simulink model "VehicleDynamics3D"  (R2017a)
settings: Solver=ode15s  StartTime=0.0  StopTime=StopTime  FixedStep=.001  MaxStep=maxStep  RelTol=relTol  AbsTol=absTol  EnableMultiTasking=on
PreLoadFcn:
  | VehicleDynamicsInitialization
model workspace: external: MATLAB File sm_suspension_templates_params.m (data not in the file)
values from neighbouring files (symbols this model uses):
  followerCameraX = 7.5    [VehicleDynamicsInitialization.m]
  followerCameraZ = 3    [VehicleDynamicsInitialization.m]
  frontCameraX = -1.75    [VehicleDynamicsInitialization.m]
  frontCameraZ = 0.35    [VehicleDynamicsInitialization.m]
  isoCameraAimX = (1/2)*wheelbase    (= 0.75)    [VehicleDynamicsInitialization.m]
  isoCameraX = -3.1    [VehicleDynamicsInitialization.m]
  isoCameraY = 3.5    [VehicleDynamicsInitialization.m]
  isoCameraZ = 1.5    [VehicleDynamicsInitialization.m]
  Load = 200    [VehicleDynamicsInitialization.m]
  maxSteeringDisplacement = 10    [VehicleDynamicsInitialization.m]
  minSteeringDisplacement = -10    [VehicleDynamicsInitialization.m]
  SetPaceSampleTime = 0.1    [VehicleDynamicsInitialization.m]
  steeringInput = 0    [VehicleDynamicsInitialization.m]
  vehicleSpeed_kph = 0    [VehicleDynamicsInitialization.m]
  wheelbase = 1.5    [VehicleDynamicsInitialization.m]
undefined symbols (not defined in the file or in its folder): dwb, Floor, sigbuilder_block, wheel, X, Y, Z
libraries: sm_lib x195, sm_suspension_templates_lib x34, nesl_utility x15, Contact_Forces_Lib x4, simulink x2, fl_lib x1, aerolibanimutils x1
(part 5 of 7)

== system VehicleDynamics3D/RearSuspension/L Spr-Damp Assm ==
  Cyl Bracket : sm_suspension_templates_lib/Single Bracket  L=Lb  W=Wb  T=Tb  Rh=Rbh  rho=rho  clr=cclr
  Cyl Bracket XForm : sm_lib/Frames and Transforms/Rigid Transform  TranslationMethod=StandardAxis  TranslationStandardOffset=Lc/2  TranslationLengthUnit=cm  TranslationStandardAxis=-Z  TranslationCartesianOffset=[0 0 0]  TranslationROffset=0  TranslationROffsetUnits=m  TranslationZOffset=0  TranslationZOffsetUnits=m  TranslationThetaOffset=0  TranslationThetaOffsetUnits=deg  RotationMethod=AlignedAxes  RotationAngleUnits=deg  RotationStandardAxis=+Z  RotationAngle=0  RotationArbitraryAxis=[0 0 1]  FollAlignAxisA=+Z  BaseAlignAxisA=-Z  FollAlignAxisB=+X  BaseAlignAxisB=-X  RotationSequenceAxes=FollowerAxes  RotationSequence=XYX  RotationSequenceAngles=[0 0 0]  RotationSequenceAnglesUnits=deg  RotationMatrix=[1 0 0; 0 1 0; 0 0 1]
  Cyl-Piston Joint : sm_lib/Joints/Prismatic Joint  SenseConstraintForce=off  SenseConstraintForceX=off  SenseConstraintForceY=off  SenseConstraintForceZ=off  SenseConstraintTorque=off  SenseConstraintTorqueX=off  SenseConstraintTorqueY=off  SenseConstraintTorqueZ=off  SenseTotalForce=off  SenseTotalForceX=off  SenseTotalForceY=off  SenseTotalForceZ=off  SenseTotalTorque=off  SenseTotalTorqueX=off  SenseTotalTorqueY=off  SenseTotalTorqueZ=off  CompositeWrenchDir=FollowerOnBase  CompositeWrenchFrame=BaseFrame  EquilibriumPosition=Ls-(Lc-Lp)/2  EquilibriumPositionUnits=cm  SpringStiffness=Ks  SpringStiffnessUnits=N/m  DampingCoefficient=Kb  DampingCoefficientUnits=N/(m/s)  TorqueActuationMode=NoTorque  MotionActuationMode=ComputedMotion  SensePosition=on  SenseVelocity=off  SenseAcceleration=off  SenseTorqueForce=off  PositionTargetSpecify=off  PositionTargetPriority=Low  PositionTargetValue=Lp/2  PositionTargetValueUnits=cm  VelocityTargetSpecify=off  VelocityTargetPriority=High  VelocityTargetValue=0  VelocityTargetValueUnits=m/s
  Cylinder : sm_lib/Body Elements/Solid  InertiaType=CalculateFromGeometry  Mass=1  MassUnits=kg  CenterOfMass=[0 0 0]  CenterOfMassUnits=m  MomentsOfInertia=[1 1 1]  MomentsOfInertiaUnits=kg*m^2  ProductsOfInertia=[0 0 0]  ProductsOfInertiaUnits=kg*m^2  DensityBased=on  Density=rho  DensityUnits=kg/(m^3)  DoExposeReferenceFrame=on  SerializedFrames=<Frames/>  GraphicType=FromGeometry  MarkerShape=Sphere  MarkerSize=10  MarkerSizeUnits=m  GraphicVisPropType=SimpleVisualProperties  GraphicDiffuseColor=cclr  GraphicSpecularColor=[0.5 0.5 0.5 1.0]  GraphicAmbientColor=[0.15 0.15 0.15 1.0]  GraphicEmissiveColor=[0.0 0.0 0.0 1.0]  GraphicShininess=75  GraphicOpacity=0.75  GeometryShape=GeneralSolidOfRevolution  RectangleSize=[1 1]  RectangleSizeUnits=m  BrickDimensions=[1 1 1]  BrickDimensionUnits=m  CylinderRadius=1  CylinderRadiusUnits=m  CylinderLength=1  CylinderLengthUnits=m  SphereRadius=1  SphereRadiusUnits=m  EllipsoidRadii=[1 1 1]  EllipsoidRadiiUnits=m  ExtrusionCrossSection=[1 1; -1 1; -1 -1; 1 -1]  ExtrusionCrossSectionUnits=m  ExtrusionLength=1  ExtrusionLengthUnits=m  PolygonNumSides=3  PolygonOuterRadius=1  PolygonOuterRadiusUnits=m  ExtGeomFileType=STL  ExtGeomFileUnits=m  RevolutionCrossSection=cyl_xsec  RevolutionCrossSectionUnits=cm  RevolutionExtent=Full  RevolutionAngle=180  RevolutionAngleUnits=deg
  PS-Simulink Converter : nesl_utility/PS-Simulink Converter  PhysicalDomain=network_engine_domain  SubClassName=ps_output  LeftPortType=input  RightPortType=output  PseudoPeriodic=off  Frequencies=[]  Unit=cm  AffineConversion=off
  Pistion Bracket : sm_suspension_templates_lib/Single Bracket  L=Lb  W=Wb  T=Tb  Rh=Rbh  rho=rho  clr=pclr
  Piston : sm_lib/Body Elements/Solid  InertiaType=CalculateFromGeometry  Mass=1  MassUnits=kg  CenterOfMass=[0 0 0]  CenterOfMassUnits=m  MomentsOfInertia=[1 1 1]  MomentsOfInertiaUnits=kg*m^2  ProductsOfInertia=[0 0 0]  ProductsOfInertiaUnits=kg*m^2  DensityBased=on  Density=rho  DensityUnits=kg/(m^3)  DoExposeReferenceFrame=on  SerializedFrames=<Frames/>  GraphicType=FromGeometry  MarkerShape=Sphere  MarkerSize=10  MarkerSizeUnits=m  GraphicVisPropType=SimpleVisualProperties  GraphicDiffuseColor=pclr  GraphicSpecularColor=[0.5 0.5 0.5 1.0]  GraphicAmbientColor=[0.15 0.15 0.15 1.0]  GraphicEmissiveColor=[0.0 0.0 0.0 1.0]  GraphicShininess=75  GraphicOpacity=1  GeometryShape=GeneralSolidOfRevolution  RectangleSize=[1 1]  RectangleSizeUnits=m  BrickDimensions=[1 1 1]  BrickDimensionUnits=m  CylinderRadius=1  CylinderRadiusUnits=m  CylinderLength=1  CylinderLengthUnits=m  SphereRadius=1  SphereRadiusUnits=m  EllipsoidRadii=[1 1 1]  EllipsoidRadiiUnits=m  ExtrusionCrossSection=[1 1; -1 1; -1 -1; 1 -1]  ExtrusionCrossSectionUnits=m  ExtrusionLength=1  ExtrusionLengthUnits=m  PolygonNumSides=3  PolygonOuterRadius=1  PolygonOuterRadiusUnits=m  ExtGeomFileType=STL  ExtGeomFileUnits=m  RevolutionCrossSection=piston_xsec  RevolutionCrossSectionUnits=cm  RevolutionExtent=Full  RevolutionAngle=180  RevolutionAngleUnits=deg
  Piston Bracket XForm : sm_lib/Frames and Transforms/Rigid Transform  TranslationMethod=StandardAxis  TranslationStandardOffset=Lp/2  TranslationLengthUnit=cm  TranslationStandardAxis=+Z  TranslationCartesianOffset=[0 0 0]  TranslationROffset=0  TranslationROffsetUnits=m  TranslationZOffset=0  TranslationZOffsetUnits=m  TranslationThetaOffset=0  TranslationThetaOffsetUnits=deg  RotationMethod=None  RotationAngleUnits=deg  RotationStandardAxis=+Z  RotationAngle=0  RotationArbitraryAxis=[0 0 1]  FollAlignAxisA=+Z  BaseAlignAxisA=+Z  FollAlignAxisB=+X  BaseAlignAxisB=-X  RotationSequenceAxes=FollowerAxes  RotationSequence=XYX  RotationSequenceAngles=[0 0 0]  RotationSequenceAnglesUnits=deg  RotationMatrix=[1 0 0; 0 1 0; 0 0 1]
  Terminator : Terminator
  P : PMIOPort  Port=1  Side=Right
  C : PMIOPort  Port=2  Side=Left
  wires:
  PS-Simulink Converter/1 -> Terminator/1  "RLSuspensionTravel_cm"
  connections:
  C/RConn1 -- Cyl Bracket/LConn1
  Pistion Bracket/LConn1 -- P/RConn1
  Pistion Bracket/RConn1 -- Piston Bracket XForm/RConn1
  Cyl Bracket/RConn1 -- Cyl Bracket XForm/RConn1
  Cyl-Piston Joint/RConn1 -- Piston/RConn1 -- Piston Bracket XForm/LConn1
  Cylinder/RConn1 -- Cyl-Piston Joint/LConn1 -- Cyl Bracket XForm/LConn1
  Cyl-Piston Joint/RConn2 -- PS-Simulink Converter/LConn1

== system VehicleDynamics3D/RearSuspension/L Suspension Assembly ==
  Knuckle : Subsystem  mask(Steering knuckle){H=dwb.knuckle.height, L=dwb.knuckle.length, T=dwb.knuckle.thickness, Wpr=dwb.knuckle.wheelattachprojwidth, Hpr=dwb.knuckle.wheelattachprojheight, Wc=dwb.knuckle.wishboneconnectorwidth, Rd=dwb.knuckle.driveshaftradius, Hd=dwb.knuckle.driveshaftheight, Rr=dwb.knuckle.chamferradius, Rt=dwb.knuckle.transitionradius, Rb=dwb.knuckle.ball.radius, Rp=dwb.knuckle.pin.radius, Hp=dwb.knuckle.pin.height, Ls=dwb.knuckle.steerarm.length, Ws=dwb.knuckle.steerarm.width, Ts=dwb.knuckle.steerarm.thickness, Hsf=dwb.knuckle.steerarm.forkheight, Lsf=dwb.knuckle.steerarm.forklength, Osf=dwb.knuckle.steerarm.forkoffset, Rsp=dwb.knuckle.pinradius, Rsr=dwb.knuckle.chamferradius, Rev=on, rho=dwb.knuckle.density, clr=dwb.knuckle.color}
      mask prompts: H "Height (cm):"; L "Length (cm):"; T "Thickness (cm):"; Wpr "Width of wheel attach projection (cm):"; Hpr "Height of wheel attach projection (cm):"; Wc "Width of wishbone connectors (cm):"; Rd "Drive shaft hole radius (cm):"; Hd "Drive shaft bearing housing height (cm):"; Rr "Chamfer/fillet radius (cm):"; Rt "Transition radius to wheel attach projection (cm):"; Rb "Ball radius (cm):"; Rp "Pin radius (cm):"; Hp "Pin height (cm):"; Ls "Length of arm (cm):"; Ws "Width of arm (cm):"; Ts "Thickness of arm (cm):"; Hsf "Height of forked section (cm):"; Lsf "Length of forked section (cm):"; Osf "Offset of forked section (cm):"; Rsp "Pin radius (cm):"; Rsr "Chamfer/fillet radius (cm):"; Rev "Reverse direction:"; rho "Density (kg/m^3):"; clr "Color ([r g b]):"
      mask help: This block models a steering knuckle. The wheel hub attaches to the steering knuckle. The steering knuckle attaches to the wishbone links. The ports U and D correspond to the frames where the knuckle connects to the wishbone links. The port W corresponds to the frame where the wheel hub attaches to the knuckle. The knuckle also has a rigidly attached steering arm that attaches to the steering rack via tie rods. The port S corresponds to the frame where the steering arm attaches to the tie rod.
      mask init:
      | s_knuckle_xsec = [0 -Hd/2; 0 -Hpr/2; Wpr -Hpr/2; Wpr -H/2;
      |                 Wpr+Wc -H/2; Wpr+Wc -H/2+T; Wpr+T -H/2+T;
      |                  Wpr+T -Hd/2];
      | 
      | s_knuckle_xsec = simmechanics.demohelpers.round_corners(s_knuckle_xsec, 2:7, ...
      |                              [Rr Rt Rr*ones(1,4)], 20);
      | 
      | n_knuckle_xsec = flipud([s_knuckle_xsec(:,1) -s_knuckle_xsec(:,2)]);                         
      | 
      | Roh = sqrt((L/2)^2 + (Hd/2)^2);
      | phi = atan2(Hd,L);
      | theta = linspace(pi/2-phi,pi/2+phi,50)';
      | sh_xsec = [Roh*cos(theta) Roh*sin(theta)];
      | theta = linspace(3*pi/2-phi,3*pi/2+phi,50)';
      | sh_xsec = [sh_xsec; Roh*cos(theta) Roh*sin(theta)];
      | theta = linspace(5*pi/2-phi,pi/2-phi,100)';
      | sh_xsec = [sh_xsec; sh_xsec(1,:); Rd*cos(theta) Rd*sin(theta)];
      | 
      | % Convert Rev variable into +/- 1 instead of 0 or 1
      | sgn = (2*Rev-1);
      mask Display:
      | image(imread(fullfile(matlabroot,'toolbox','physmod','sm','smdemos','suspension_templates','images','sm_isuspension_knuckle.png')));
      | port_label('RConn',1,'U');
      | port_label('RConn',2,'D');
      | port_label('LConn',1,'W');
  Lower Wishbone : sm_suspension_templates_lib/Lower Wishbone  L1=dwb.lwb.longlength  L2=dwb.lwb.shortlength  L3=dwb.lwb.wheellinklength  W3=dwb.lwb.wheellinkwidth  W=dwb.lwb.width  T=dwb.lwb.thickness  Rb=dwb.lwb.baseradius  Ob=dwb.lwb.basearcoffset  Rev=on  Lb=dwb.lwb.bracket.length  Rsh=dwb.lwb.bracket.radius  Rs=dwb.lwb.socket.radius  Hi=dwb.lwb.socket.height  Rh=dwb.lwb.socket.holeradius  Oh=dwb.lwb.socket.holeoffset  Odb=dwb.lwb.damperbracket.offset  Wdb=dwb.lwb.damperbracket.width  Ldb=dwb.lwb.damperbracket.length  Tdb=dwb.lwb.damperbracket.thickness  Sdb=dwb.lwb.damperbracket.spacing  Rhdb=dwb.lwb.damperbracket.holeradius  rho=dwb.lwb.density  clr=dwb.lwb.color
  SW Damp Joint : sm_lib/Joints/Revolute Joint  SenseConstraintForce=off  SenseConstraintForceX=off  SenseConstraintForceY=off  SenseConstraintForceZ=off  SenseConstraintTorque=off  SenseConstraintTorqueX=off  SenseConstraintTorqueY=off  SenseConstraintTorqueZ=off  SenseTotalForce=off  SenseTotalForceX=off  SenseTotalForceY=off  SenseTotalForceZ=off  SenseTotalTorque=off  SenseTotalTorqueX=off  SenseTotalTorqueY=off  SenseTotalTorqueZ=off  CompositeWrenchDir=FollowerOnBase  CompositeWrenchFrame=BaseFrame  EquilibriumPosition=0  EquilibriumPositionUnits=deg  SpringStiffness=0  SpringStiffnessUnits=N*m/deg  DampingCoefficient=0  DampingCoefficientUnits=N*m/(deg/s)  TorqueActuationMode=NoTorque  MotionActuationMode=ComputedMotion  SensePosition=off  SenseVelocity=off  SenseAcceleration=off  SenseTorqueForce=off  PositionTargetSpecify=off  PositionTargetPriority=Low  PositionTargetValue=-30  PositionTargetValueUnits=deg  VelocityTargetSpecify=off  VelocityTargetPriority=High  VelocityTargetValue=0  VelocityTargetValueUnits=deg/s
  Subsystem : Subsystem
  Subsystem1 : Subsystem
  Upper Wishbone : sm_suspension_templates_lib/Wishbone  L1=dwb.uwb.longlength  L2=dwb.uwb.shortlength  L3=dwb.uwb.wheellinklength  W3=dwb.uwb.wheellinkwidth  W=dwb.uwb.width  T=dwb.uwb.thickness  Rb=dwb.uwb.baseradius  Ob=dwb.uwb.basearcoffset  Rev=on  Lb=dwb.uwb.bracket.length  Rsh=dwb.uwb.bracket.radius  Rs=dwb.uwb.socket.radius  Hi=dwb.uwb.socket.height  Rh=dwb.uwb.socket.ballradius  Oh=dwb.uwb.socket.offset  rho=dwb.uwb.density  clr=dwb.uwb.color
  UA : PMIOPort  Port=1  Side=Right
  UB : PMIOPort  Port=2  Side=Right
  T : PMIOPort  Port=3  Side=Left
  DP : PMIOPort  Port=4  Side=Right
  DA : PMIOPort  Port=5  Side=Right
  DB : PMIOPort  Port=6  Side=Right
  connections:
  Lower Wishbone/RConn1 -- Subsystem1/RConn1
  Knuckle/LConn1 -- T/RConn1
  Lower Wishbone/LConn3 -- DB/RConn1
  Lower Wishbone/LConn2 -- DA/RConn1
  Upper Wishbone/LConn1 -- UA/RConn1
  UB/RConn1 -- Upper Wishbone/LConn2
  Knuckle/RConn2 -- Subsystem1/LConn1
  SW Damp Joint/LConn1 -- Lower Wishbone/LConn1
  SW Damp Joint/RConn1 -- DP/RConn1
  Upper Wishbone/RConn1 -- Subsystem/RConn1
  Knuckle/RConn1 -- Subsystem/LConn1

== system VehicleDynamics3D/RearSuspension/R Spr-Damp Assm ==
  Cyl Bracket : sm_suspension_templates_lib/Single Bracket  L=Lb  W=Wb  T=Tb  Rh=Rbh  rho=rho  clr=cclr
  Cyl Bracket XForm : sm_lib/Frames and Transforms/Rigid Transform  TranslationMethod=StandardAxis  TranslationStandardOffset=Lc/2  TranslationLengthUnit=cm  TranslationStandardAxis=-Z  TranslationCartesianOffset=[0 0 0]  TranslationROffset=0  TranslationROffsetUnits=m  TranslationZOffset=0  TranslationZOffsetUnits=m  TranslationThetaOffset=0  TranslationThetaOffsetUnits=deg  RotationMethod=AlignedAxes  RotationAngleUnits=deg  RotationStandardAxis=+Z  RotationAngle=0  RotationArbitraryAxis=[0 0 1]  FollAlignAxisA=+Z  BaseAlignAxisA=-Z  FollAlignAxisB=+X  BaseAlignAxisB=-X  RotationSequenceAxes=FollowerAxes  RotationSequence=XYX  RotationSequenceAngles=[0 0 0]  RotationSequenceAnglesUnits=deg  RotationMatrix=[1 0 0; 0 1 0; 0 0 1]
  Cyl-Piston Joint : sm_lib/Joints/Prismatic Joint  SenseConstraintForce=off  SenseConstraintForceX=off  SenseConstraintForceY=off  SenseConstraintForceZ=off  SenseConstraintTorque=off  SenseConstraintTorqueX=off  SenseConstraintTorqueY=off  SenseConstraintTorqueZ=off  SenseTotalForce=off  SenseTotalForceX=off  SenseTotalForceY=off  SenseTotalForceZ=off  SenseTotalTorque=off  SenseTotalTorqueX=off  SenseTotalTorqueY=off  SenseTotalTorqueZ=off  CompositeWrenchDir=FollowerOnBase  CompositeWrenchFrame=BaseFrame  EquilibriumPosition=Ls-(Lc-Lp)/2  EquilibriumPositionUnits=cm  SpringStiffness=Ks  SpringStiffnessUnits=N/m  DampingCoefficient=Kb  DampingCoefficientUnits=N/(m/s)  TorqueActuationMode=NoTorque  MotionActuationMode=ComputedMotion  SensePosition=on  SenseVelocity=off  SenseAcceleration=off  SenseTorqueForce=off  PositionTargetSpecify=off  PositionTargetPriority=Low  PositionTargetValue=Lp/2  PositionTargetValueUnits=cm  VelocityTargetSpecify=off  VelocityTargetPriority=High  VelocityTargetValue=0  VelocityTargetValueUnits=m/s
  Cylinder : sm_lib/Body Elements/Solid  InertiaType=CalculateFromGeometry  Mass=1  MassUnits=kg  CenterOfMass=[0 0 0]  CenterOfMassUnits=m  MomentsOfInertia=[1 1 1]  MomentsOfInertiaUnits=kg*m^2  ProductsOfInertia=[0 0 0]  ProductsOfInertiaUnits=kg*m^2  DensityBased=on  Density=rho  DensityUnits=kg/(m^3)  DoExposeReferenceFrame=on  SerializedFrames=<Frames/>  GraphicType=FromGeometry  MarkerShape=Sphere  MarkerSize=10  MarkerSizeUnits=m  GraphicVisPropType=SimpleVisualProperties  GraphicDiffuseColor=cclr  GraphicSpecularColor=[0.5 0.5 0.5 1.0]  GraphicAmbientColor=[0.15 0.15 0.15 1.0]  GraphicEmissiveColor=[0.0 0.0 0.0 1.0]  GraphicShininess=75  GraphicOpacity=0.75  GeometryShape=GeneralSolidOfRevolution  RectangleSize=[1 1]  RectangleSizeUnits=m  BrickDimensions=[1 1 1]  BrickDimensionUnits=m  CylinderRadius=1  CylinderRadiusUnits=m  CylinderLength=1  CylinderLengthUnits=m  SphereRadius=1  SphereRadiusUnits=m  EllipsoidRadii=[1 1 1]  EllipsoidRadiiUnits=m  ExtrusionCrossSection=[1 1; -1 1; -1 -1; 1 -1]  ExtrusionCrossSectionUnits=m  ExtrusionLength=1  ExtrusionLengthUnits=m  PolygonNumSides=3  PolygonOuterRadius=1  PolygonOuterRadiusUnits=m  ExtGeomFileType=STL  ExtGeomFileUnits=m  RevolutionCrossSection=cyl_xsec  RevolutionCrossSectionUnits=cm  RevolutionExtent=Full  RevolutionAngle=180  RevolutionAngleUnits=deg
  PS-Simulink Converter : nesl_utility/PS-Simulink Converter  PhysicalDomain=network_engine_domain  SubClassName=ps_output  LeftPortType=input  RightPortType=output  PseudoPeriodic=off  Frequencies=[]  Unit=cm  AffineConversion=off
  Pistion Bracket : sm_suspension_templates_lib/Single Bracket  L=Lb  W=Wb  T=Tb  Rh=Rbh  rho=rho  clr=pclr
  Piston : sm_lib/Body Elements/Solid  InertiaType=CalculateFromGeometry  Mass=1  MassUnits=kg  CenterOfMass=[0 0 0]  CenterOfMassUnits=m  MomentsOfInertia=[1 1 1]  MomentsOfInertiaUnits=kg*m^2  ProductsOfInertia=[0 0 0]  ProductsOfInertiaUnits=kg*m^2  DensityBased=on  Density=rho  DensityUnits=kg/(m^3)  DoExposeReferenceFrame=on  SerializedFrames=<Frames/>  GraphicType=FromGeometry  MarkerShape=Sphere  MarkerSize=10  MarkerSizeUnits=m  GraphicVisPropType=SimpleVisualProperties  GraphicDiffuseColor=pclr  GraphicSpecularColor=[0.5 0.5 0.5 1.0]  GraphicAmbientColor=[0.15 0.15 0.15 1.0]  GraphicEmissiveColor=[0.0 0.0 0.0 1.0]  GraphicShininess=75  GraphicOpacity=1  GeometryShape=GeneralSolidOfRevolution  RectangleSize=[1 1]  RectangleSizeUnits=m  BrickDimensions=[1 1 1]  BrickDimensionUnits=m  CylinderRadius=1  CylinderRadiusUnits=m  CylinderLength=1  CylinderLengthUnits=m  SphereRadius=1  SphereRadiusUnits=m  EllipsoidRadii=[1 1 1]  EllipsoidRadiiUnits=m  ExtrusionCrossSection=[1 1; -1 1; -1 -1; 1 -1]  ExtrusionCrossSectionUnits=m  ExtrusionLength=1  ExtrusionLengthUnits=m  PolygonNumSides=3  PolygonOuterRadius=1  PolygonOuterRadiusUnits=m  ExtGeomFileType=STL  ExtGeomFileUnits=m  RevolutionCrossSection=piston_xsec  RevolutionCrossSectionUnits=cm  RevolutionExtent=Full  RevolutionAngle=180  RevolutionAngleUnits=deg
  Piston Bracket XForm : sm_lib/Frames and Transforms/Rigid Transform  TranslationMethod=StandardAxis  TranslationStandardOffset=Lp/2  TranslationLengthUnit=cm  TranslationStandardAxis=+Z  TranslationCartesianOffset=[0 0 0]  TranslationROffset=0  TranslationROffsetUnits=m  TranslationZOffset=0  TranslationZOffsetUnits=m  TranslationThetaOffset=0  TranslationThetaOffsetUnits=deg  RotationMethod=None  RotationAngleUnits=deg  RotationStandardAxis=+Z  RotationAngle=0  RotationArbitraryAxis=[0 0 1]  FollAlignAxisA=+Z  BaseAlignAxisA=+Z  FollAlignAxisB=+X  BaseAlignAxisB=-X  RotationSequenceAxes=FollowerAxes  RotationSequence=XYX  RotationSequenceAngles=[0 0 0]  RotationSequenceAnglesUnits=deg  RotationMatrix=[1 0 0; 0 1 0; 0 0 1]
  Terminator : Terminator
  P : PMIOPort  Port=1  Side=Right
  C : PMIOPort  Port=2  Side=Left
  wires:
  PS-Simulink Converter/1 -> Terminator/1  "RRSuspensionTravel_cm"
  connections:
  C/RConn1 -- Cyl Bracket/LConn1
  Pistion Bracket/LConn1 -- P/RConn1
  Pistion Bracket/RConn1 -- Piston Bracket XForm/RConn1
  Cyl Bracket/RConn1 -- Cyl Bracket XForm/RConn1
  Cyl-Piston Joint/RConn1 -- Piston/RConn1 -- Piston Bracket XForm/LConn1
  Cylinder/RConn1 -- Cyl-Piston Joint/LConn1 -- Cyl Bracket XForm/LConn1
  Cyl-Piston Joint/RConn2 -- PS-Simulink Converter/LConn1

== system VehicleDynamics3D/RearSuspension/R Suspension Assembly ==
  Knuckle : Subsystem  mask(Steering knuckle){H=dwb.knuckle.height, L=dwb.knuckle.length, T=dwb.knuckle.thickness, Wpr=dwb.knuckle.wheelattachprojwidth, Hpr=dwb.knuckle.wheelattachprojheight, Wc=dwb.knuckle.wishboneconnectorwidth, Rd=dwb.knuckle.driveshaftradius, Hd=dwb.knuckle.driveshaftheight, Rr=dwb.knuckle.chamferradius, Rt=dwb.knuckle.transitionradius, Rb=dwb.knuckle.ball.radius, Rp=dwb.knuckle.pin.radius, Hp=dwb.knuckle.pin.height, Ls=dwb.knuckle.steerarm.length, Ws=dwb.knuckle.steerarm.width, Ts=dwb.knuckle.steerarm.thickness, Hsf=dwb.knuckle.steerarm.forkheight, Lsf=dwb.knuckle.steerarm.forklength, Osf=dwb.knuckle.steerarm.forkoffset, Rsp=dwb.knuckle.pinradius, Rsr=dwb.knuckle.chamferradius, Rev=off, rho=dwb.knuckle.density, clr=dwb.knuckle.color}
      mask prompts: H "Height (cm):"; L "Length (cm):"; T "Thickness (cm):"; Wpr "Width of wheel attach projection (cm):"; Hpr "Height of wheel attach projection (cm):"; Wc "Width of wishbone connectors (cm):"; Rd "Drive shaft hole radius (cm):"; Hd "Drive shaft bearing housing height (cm):"; Rr "Chamfer/fillet radius (cm):"; Rt "Transition radius to wheel attach projection (cm):"; Rb "Ball radius (cm):"; Rp "Pin radius (cm):"; Hp "Pin height (cm):"; Ls "Length of arm (cm):"; Ws "Width of arm (cm):"; Ts "Thickness of arm (cm):"; Hsf "Height of forked section (cm):"; Lsf "Length of forked section (cm):"; Osf "Offset of forked section (cm):"; Rsp "Pin radius (cm):"; Rsr "Chamfer/fillet radius (cm):"; Rev "Reverse direction:"; rho "Density (kg/m^3):"; clr "Color ([r g b]):"
      mask help: This block models a steering knuckle. The wheel hub attaches to the steering knuckle. The steering knuckle attaches to the wishbone links. The ports U and D correspond to the frames where the knuckle connects to the wishbone links. The port W corresponds to the frame where the wheel hub attaches to the knuckle. The knuckle also has a rigidly attached steering arm that attaches to the steering rack via tie rods. The port S corresponds to the frame where the steering arm attaches to the tie rod.
      mask init: same as VehicleDynamics3D/RearSuspension/L Suspension Assembly/Knuckle
      mask Display:
      | image(imread(fullfile(matlabroot,'toolbox','physmod','sm','smdemos','suspension_templates','images','sm_isuspension_knuckle.png')));
      | port_label('RConn',1,'U');
      | port_label('RConn',2,'D');
      | port_label('LConn',1,'W');
  Lower Wishbone : sm_suspension_templates_lib/Lower Wishbone  L1=dwb.lwb.longlength  L2=dwb.lwb.shortlength  L3=dwb.lwb.wheellinklength  W3=dwb.lwb.wheellinkwidth  W=dwb.lwb.width  T=dwb.lwb.thickness  Rb=dwb.lwb.baseradius  Ob=dwb.lwb.basearcoffset  Rev=off  Lb=dwb.lwb.bracket.length  Rsh=dwb.lwb.bracket.radius  Rs=dwb.lwb.socket.radius  Hi=dwb.lwb.socket.height  Rh=dwb.lwb.socket.holeradius  Oh=dwb.lwb.socket.holeoffset  Odb=dwb.lwb.damperbracket.offset  Wdb=dwb.lwb.damperbracket.width  Ldb=dwb.lwb.damperbracket.length  Tdb=dwb.lwb.damperbracket.thickness  Sdb=dwb.lwb.damperbracket.spacing  Rhdb=dwb.lwb.damperbracket.holeradius  rho=dwb.lwb.density  clr=dwb.lwb.color
  SE Damp Joint : sm_lib/Joints/Revolute Joint  SenseConstraintForce=off  SenseConstraintForceX=off  SenseConstraintForceY=off  SenseConstraintForceZ=off  SenseConstraintTorque=off  SenseConstraintTorqueX=off  SenseConstraintTorqueY=off  SenseConstraintTorqueZ=off  SenseTotalForce=off  SenseTotalForceX=off  SenseTotalForceY=off  SenseTotalForceZ=off  SenseTotalTorque=off  SenseTotalTorqueX=off  SenseTotalTorqueY=off  SenseTotalTorqueZ=off  CompositeWrenchDir=FollowerOnBase  CompositeWrenchFrame=BaseFrame  EquilibriumPosition=0  EquilibriumPositionUnits=deg  SpringStiffness=0  SpringStiffnessUnits=N*m/deg  DampingCoefficient=0  DampingCoefficientUnits=N*m/(deg/s)  TorqueActuationMode=NoTorque  MotionActuationMode=ComputedMotion  SensePosition=off  SenseVelocity=off  SenseAcceleration=off  SenseTorqueForce=off  PositionTargetSpecify=off  PositionTargetPriority=Low  PositionTargetValue=150  PositionTargetValueUnits=deg  VelocityTargetSpecify=off  VelocityTargetPriority=High  VelocityTargetValue=0  VelocityTargetValueUnits=deg/s
  Subsystem : Subsystem
  Subsystem1 : Subsystem
  Upper Wishbone : sm_suspension_templates_lib/Wishbone  L1=dwb.uwb.longlength  L2=dwb.uwb.shortlength  L3=dwb.uwb.wheellinklength  W3=dwb.uwb.wheellinkwidth  W=dwb.uwb.width  T=dwb.uwb.thickness  Rb=dwb.uwb.baseradius  Ob=dwb.uwb.basearcoffset  Rev=off  Lb=dwb.uwb.bracket.length  Rsh=dwb.uwb.bracket.radius  Rs=dwb.uwb.socket.radius  Hi=dwb.uwb.socket.height  Rh=dwb.uwb.socket.ballradius  Oh=dwb.uwb.socket.offset  rho=dwb.uwb.density  clr=dwb.uwb.color
  UA : PMIOPort  Port=1  Side=Left
  UB : PMIOPort  Port=2  Side=Left
  T : PMIOPort  Port=3  Side=Right
  DP : PMIOPort  Port=4  Side=Left
  DA : PMIOPort  Port=5  Side=Left
  DB : PMIOPort  Port=6  Side=Left
  connections:
  Lower Wishbone/RConn1 -- Subsystem/LConn1
  Lower Wishbone/LConn3 -- DB/RConn1
  Lower Wishbone/LConn2 -- DA/RConn1
  UA/RConn1 -- Upper Wishbone/LConn1
  Subsystem/RConn1 -- Knuckle/RConn2
  UB/RConn1 -- Upper Wishbone/LConn2
  DP/RConn1 -- SE Damp Joint/LConn1
  SE Damp Joint/RConn1 -- Lower Wishbone/LConn1
  T/RConn1 -- Knuckle/LConn1
  Subsystem1/RConn1 -- Knuckle/RConn1
  Subsystem1/LConn1 -- Upper Wishbone/RConn1

== system VehicleDynamics3D/WheelFL/FrontLeftWeelContact ==
  Bus Selector : BusSelector  OutputSignals=Normal Force,Friction Force
  Math Function : Math  Operator=square  SaturateOnIntegerOverflow=on
  Rigid Transform : sm_lib/Frames and Transforms/Rigid Transform  TranslationMethod=StandardAxis  TranslationStandardOffset=-wheel.tire.outerradius*.01  TranslationLengthUnit=m  TranslationStandardAxis=+Z  TranslationCartesianOffset=[0 0 0]  TranslationROffset=0  TranslationROffsetUnits=m  TranslationZOffset=0  TranslationZOffsetUnits=m  TranslationThetaOffset=0  TranslationThetaOffsetUnits=deg  RotationMethod=None  RotationAngleUnits=deg  RotationStandardAxis=+Z  RotationAngle=0  RotationArbitraryAxis=[0 0 1]  FollAlignAxisA=+X  BaseAlignAxisA=-X  FollAlignAxisB=+Z  BaseAlignAxisB=+Z  RotationSequenceAxes=FollowerAxes  RotationSequence=XYX  RotationSequenceAngles=[0 0 0]  RotationSequenceAnglesUnits=deg  RotationMatrix=[1 0 0; 0 1 0; 0 0 1]
  Signal Conversion : SignalConversion  OverrideOpt=off
  Signal Conversion1 : SignalConversion  OverrideOpt=off
  Sphere to Plane Force : Contact_Forces_Lib/3D/Sphere to Plane Force  sphere_rad=wheel.tire.outerradius*.01  plane_lenx=Floor.l  plane_leny=Floor.w  plane_depth=Floor.h/2  force_law=Nonlinear  k_contact=contactStiffness  b_contact=contactDamping  pen_full_damp_F=1e-4  pen_exponent=1  custom_param_1=1  custom_param_2=1  friction_law=Stick-Slip Continuous  mu_kinetic=kineticFrictionCoeff  mu_static=staticFrictionCoeff  v_thr=velocityThreshold  vis_on=off  vis_opc_en=0  vis_len_plaBz=0.005  vis_clr=[0.9 0.2 0.2]  vis_opc=0.7
  Sqrt : Sqrt  SaturateOnIntegerOverflow=on
  Sum of Elements : Sum  Inputs=+
  Terminator : Terminator
  Terminator1 : Terminator
  Conn1 : PMIOPort  Port=1  Side=Right
  Conn2 : PMIOPort  Port=2  Side=Left
  wires:
  Sphere to Plane Force/1 -> Bus Selector/1  "FrontLeft"
  Math Function/1 -> Sum of Elements/1
  Sum of Elements/1 -> Sqrt/1
  Bus Selector/2 -> Math Function/1  "<Friction Force>"
  Bus Selector/1 -> Signal Conversion/1  "<Normal Force>"
  Sqrt/1 -> Signal Conversion1/1
  Signal Conversion/1 -> Terminator/1  "FrontLeftTireLoad"
  Signal Conversion1/1 -> Terminator1/1  "FrontLeftFriction"
  connections:
  Conn2/RConn1 -- Sphere to Plane Force/RConn1
  Sphere to Plane Force/LConn1 -- Rigid Transform/LConn1
  Conn1/RConn1 -- Rigid Transform/RConn1

== system VehicleDynamics3D/WheelFR/FrontRightWeelContact ==
  Bus Selector : BusSelector  OutputSignals=Normal Force,Friction Force
  Math Function : Math  Operator=square  SaturateOnIntegerOverflow=on
  Rigid Transform : sm_lib/Frames and Transforms/Rigid Transform  TranslationMethod=StandardAxis  TranslationStandardOffset=-wheel.tire.outerradius*.01  TranslationLengthUnit=m  TranslationStandardAxis=+Z  TranslationCartesianOffset=[0 0 0]  TranslationROffset=0  TranslationROffsetUnits=m  TranslationZOffset=0  TranslationZOffsetUnits=m  TranslationThetaOffset=0  TranslationThetaOffsetUnits=deg  RotationMethod=None  RotationAngleUnits=deg  RotationStandardAxis=+Z  RotationAngle=0  RotationArbitraryAxis=[0 0 1]  FollAlignAxisA=+X  BaseAlignAxisA=-X  FollAlignAxisB=+Z  BaseAlignAxisB=+Z  RotationSequenceAxes=FollowerAxes  RotationSequence=XYX  RotationSequenceAngles=[0 0 0]  RotationSequenceAnglesUnits=deg  RotationMatrix=[1 0 0; 0 1 0; 0 0 1]
  Signal Conversion : SignalConversion  OverrideOpt=off
  Signal Conversion1 : SignalConversion  OverrideOpt=off
  Sphere to Plane Force : Contact_Forces_Lib/3D/Sphere to Plane Force  sphere_rad=wheel.tire.outerradius*.01  plane_lenx=Floor.l  plane_leny=Floor.w  plane_depth=Floor.h/2  force_law=Linear  k_contact=contactStiffness  b_contact=contactDamping  pen_full_damp_F=1e-4  pen_exponent=1  custom_param_1=1  custom_param_2=1  friction_law=Stick-Slip Continuous  mu_kinetic=kineticFrictionCoeff  mu_static=staticFrictionCoeff  v_thr=velocityThreshold  vis_on=off  vis_opc_en=0  vis_len_plaBz=0.005  vis_clr=[0.9 0.2 0.2]  vis_opc=0.7
  Sqrt : Sqrt  SaturateOnIntegerOverflow=on
  Sum of Elements : Sum  Inputs=+
  Terminator : Terminator
  Terminator1 : Terminator
  Conn1 : PMIOPort  Port=1  Side=Right
  Conn2 : PMIOPort  Port=2  Side=Left
  wires:
  Sphere to Plane Force/1 -> Bus Selector/1  "FrontRight"
  Signal Conversion1/1 -> Terminator1/1  "FrontRightFriction"
  Bus Selector/1 -> Signal Conversion/1  "<Normal Force>"
  Sum of Elements/1 -> Sqrt/1
  Signal Conversion/1 -> Terminator/1  "FrontRightTireLoad"
  Math Function/1 -> Sum of Elements/1
  Bus Selector/2 -> Math Function/1  "<Friction Force>"
  Sqrt/1 -> Signal Conversion1/1
  connections:
  Conn1/RConn1 -- Rigid Transform/RConn1
  Sphere to Plane Force/LConn1 -- Rigid Transform/LConn1
  Conn2/RConn1 -- Sphere to Plane Force/RConn1

== system VehicleDynamics3D/WheelRL/RearLeftWeelContact ==
  Bus Selector : BusSelector  OutputSignals=Normal Force,Friction Force
  Math Function : Math  Operator=square  SaturateOnIntegerOverflow=on
  Rigid Transform : sm_lib/Frames and Transforms/Rigid Transform  TranslationMethod=StandardAxis  TranslationStandardOffset=-wheel.tire.outerradius*.01  TranslationLengthUnit=m  TranslationStandardAxis=+Z  TranslationCartesianOffset=[0 0 0]  TranslationROffset=0  TranslationROffsetUnits=m  TranslationZOffset=0  TranslationZOffsetUnits=m  TranslationThetaOffset=0  TranslationThetaOffsetUnits=deg  RotationMethod=None  RotationAngleUnits=deg  RotationStandardAxis=+Z  RotationAngle=0  RotationArbitraryAxis=[0 0 1]  FollAlignAxisA=+X  BaseAlignAxisA=-X  FollAlignAxisB=+Z  BaseAlignAxisB=+Z  RotationSequenceAxes=FollowerAxes  RotationSequence=XYX  RotationSequenceAngles=[0 0 0]  RotationSequenceAnglesUnits=deg  RotationMatrix=[1 0 0; 0 1 0; 0 0 1]
  Signal Conversion : SignalConversion  OverrideOpt=off
  Signal Conversion1 : SignalConversion  OverrideOpt=off
  Sphere to Plane Force : Contact_Forces_Lib/3D/Sphere to Plane Force  sphere_rad=wheel.tire.outerradius*.01  plane_lenx=Floor.l  plane_leny=Floor.w  plane_depth=Floor.h/2  force_law=Linear  k_contact=contactStiffness  b_contact=contactDamping  pen_full_damp_F=1e-4  pen_exponent=1  custom_param_1=1  custom_param_2=1  friction_law=Stick-Slip Continuous  mu_kinetic=kineticFrictionCoeff  mu_static=staticFrictionCoeff  v_thr=velocityThreshold  vis_on=off  vis_opc_en=0  vis_len_plaBz=0.005  vis_clr=[0.9 0.2 0.2]  vis_opc=0.7
  Sqrt : Sqrt  SaturateOnIntegerOverflow=on
  Sum of Elements : Sum  Inputs=+
  Terminator : Terminator
  Terminator2 : Terminator
  Conn1 : PMIOPort  Port=1  Side=Right
  Conn2 : PMIOPort  Port=2  Side=Left
  wires:
  Sphere to Plane Force/1 -> Bus Selector/1
  Signal Conversion1/1 -> Terminator2/1  "RearLeftFriction"
  Sum of Elements/1 -> Sqrt/1
  Bus Selector/1 -> Signal Conversion/1  "<Normal Force>"
  Bus Selector/2 -> Math Function/1  "<Friction Force>"
  Signal Conversion/1 -> Terminator/1  "RearLeftTireLoad"
  Math Function/1 -> Sum of Elements/1
  Sqrt/1 -> Signal Conversion1/1
  connections:
  Conn1/RConn1 -- Rigid Transform/RConn1
  Sphere to Plane Force/LConn1 -- Rigid Transform/LConn1
  Sphere to Plane Force/RConn1 -- Conn2/RConn1

== system VehicleDynamics3D/WheelRR/RearRightWeelContact ==
  Bus Selector : BusSelector  OutputSignals=Normal Force,Friction Force
  Math Function : Math  Operator=square  SaturateOnIntegerOverflow=on
  Rigid Transform : sm_lib/Frames and Transforms/Rigid Transform  TranslationMethod=StandardAxis  TranslationStandardOffset=-wheel.tire.outerradius*.01  TranslationLengthUnit=m  TranslationStandardAxis=+Z  TranslationCartesianOffset=[0 0 0]  TranslationROffset=0  TranslationROffsetUnits=m  TranslationZOffset=0  TranslationZOffsetUnits=m  TranslationThetaOffset=0  TranslationThetaOffsetUnits=deg  RotationMethod=None  RotationAngleUnits=deg  RotationStandardAxis=+Z  RotationAngle=0  RotationArbitraryAxis=[0 0 1]  FollAlignAxisA=+X  BaseAlignAxisA=-X  FollAlignAxisB=+Z  BaseAlignAxisB=+Z  RotationSequenceAxes=FollowerAxes  RotationSequence=XYX  RotationSequenceAngles=[0 0 0]  RotationSequenceAnglesUnits=deg  RotationMatrix=[1 0 0; 0 1 0; 0 0 1]
  Signal Conversion : SignalConversion  OverrideOpt=off
  Signal Conversion1 : SignalConversion  OverrideOpt=off
  Sphere to Plane Force : Contact_Forces_Lib/3D/Sphere to Plane Force  sphere_rad=wheel.tire.outerradius*.01  plane_lenx=Floor.l  plane_leny=Floor.w  plane_depth=Floor.h/2  force_law=Linear  k_contact=contactStiffness  b_contact=contactDamping  pen_full_damp_F=1e-4  pen_exponent=1  custom_param_1=1  custom_param_2=1  friction_law=Stick-Slip Continuous  mu_kinetic=kineticFrictionCoeff  mu_static=staticFrictionCoeff  v_thr=velocityThreshold  vis_on=off  vis_opc_en=0  vis_len_plaBz=0.005  vis_clr=[0.9 0.2 0.2]  vis_opc=0.7
  Sqrt : Sqrt  SaturateOnIntegerOverflow=on
  Sum of Elements : Sum  Inputs=+
  Terminator1 : Terminator
  Terminator2 : Terminator
  Conn1 : PMIOPort  Port=1  Side=Right
  Conn2 : PMIOPort  Port=2  Side=Left
  wires:
  Sphere to Plane Force/1 -> Bus Selector/1  "RearRight"
  Bus Selector/1 -> Signal Conversion1/1  "<Normal Force>"
  Bus Selector/2 -> Signal Conversion/1  "<Friction Force>"
  Math Function/1 -> Sum of Elements/1
  Sum of Elements/1 -> Sqrt/1
  Sqrt/1 -> Terminator2/1  "RearRightFriction"
  Signal Conversion/1 -> Math Function/1
  Signal Conversion1/1 -> Terminator1/1  "RearRightTireLoad"
  connections:
  Sphere to Plane Force/LConn1 -- Rigid Transform/LConn1
  Conn1/RConn1 -- Rigid Transform/RConn1
  Conn2/RConn1 -- Sphere to Plane Force/RConn1

== system VehicleDynamics3D/FrontSuspension/6DOF Motion/WraptTo180 ==
  Yaw : Inport
  Bias : Bias  Bias=-180
  Bias1 : Bias  Bias=180
  Constant : Constant  Value=360
  Interval Test : simulink/Logic and Bit Operations/Interval Test  IntervalClosedRight=on  uplimit=180  IntervalClosedLeft=off  lowlimit=-180  OutDataTypeStr=boolean
  Math Function : Math  Operator=mod  SaturateOnIntegerOverflow=on
  Switch : Switch  Criteria=u2 ~= 0
  NormalizedYaw : Outport
  wires:
  Bias1/1 -> Math Function/1
  Switch/1 -> NormalizedYaw/1  "VehicleYawNormalized_Deg"
  Constant/1 -> Math Function/2
  Interval Test/1 -> Switch/2
  Math Function/1 -> Bias/1
  Bias/1 -> Switch/3
  Yaw/1 -> Switch/1, Interval Test/1, Bias1/1

== system VehicleDynamics3D/FrontSuspension/Chassis Assembly/Front Frame ==
  DL XForm : sm_lib/Frames and Transforms/Rigid Transform  TranslationMethod=Cartesian  TranslationStandardOffset=0  TranslationLengthUnit=cm  TranslationStandardAxis=+Z  TranslationCartesianOffset=[swc 0]  TranslationROffset=0  TranslationROffsetUnits=m  TranslationZOffset=0  TranslationZOffsetUnits=m  TranslationThetaOffset=0  TranslationThetaOffsetUnits=deg  RotationMethod=None  RotationAngleUnits=deg  RotationStandardAxis=+Z  RotationAngle=0  RotationArbitraryAxis=[0 0 1]  FollAlignAxisA=+X  BaseAlignAxisA=-X  FollAlignAxisB=+Y  BaseAlignAxisB=-Y  RotationSequenceAxes=FollowerAxes  RotationSequence=XYX  RotationSequenceAngles=[0 0 0]  RotationSequenceAnglesUnits=deg  RotationMatrix=[1 0 0; 0 1 0; 0 0 1]
  DR XForm : sm_lib/Frames and Transforms/Rigid Transform  TranslationMethod=Cartesian  TranslationStandardOffset=0  TranslationLengthUnit=cm  TranslationStandardAxis=+Z  TranslationCartesianOffset=[sec 0]  TranslationROffset=0  TranslationROffsetUnits=m  TranslationZOffset=0  TranslationZOffsetUnits=m  TranslationThetaOffset=0  TranslationThetaOffsetUnits=deg  RotationMethod=None  RotationAngleUnits=deg  RotationStandardAxis=+Z  RotationAngle=0  RotationArbitraryAxis=[0 0 1]  FollAlignAxisA=+X  BaseAlignAxisA=+Y  FollAlignAxisB=+Y  BaseAlignAxisB=+Z  RotationSequenceAxes=FollowerAxes  RotationSequence=XYX  RotationSequenceAngles=[0 0 0]  RotationSequenceAnglesUnits=deg  RotationMatrix=[1 0 0; 0 1 0; 0 0 1]
  Frame : sm_lib/Body Elements/Solid  InertiaType=CalculateFromGeometry  Mass=1  MassUnits=kg  CenterOfMass=[0 0 0]  CenterOfMassUnits=m  MomentsOfInertia=[1 1 1]  MomentsOfInertiaUnits=kg*m^2  ProductsOfInertia=[0 0 0]  ProductsOfInertiaUnits=kg*m^2  DensityBased=on  Density=rho  DensityUnits=kg/(m^3)  DoExposeReferenceFrame=on  SerializedFrames=<Frames/>  GraphicType=FromGeometry  MarkerShape=Sphere  MarkerSize=10  MarkerSizeUnits=m  GraphicVisPropType=SimpleVisualProperties  GraphicDiffuseColor=clr  GraphicSpecularColor=[0.5 0.5 0.5 1.0]  GraphicAmbientColor=[0.15 0.15 0.15 1.0]  GraphicEmissiveColor=[0.0 0.0 0.0 1.0]  GraphicShininess=75  GraphicOpacity=1.0  GeometryShape=GeneralExtrusion  RectangleSize=[1 1]  RectangleSizeUnits=m  BrickDimensions=[1 1 1]  BrickDimensionUnits=m  CylinderRadius=1  CylinderRadiusUnits=m  CylinderLength=1  CylinderLengthUnits=m  SphereRadius=1  SphereRadiusUnits=m  EllipsoidRadii=[1 1 1]  EllipsoidRadiiUnits=m  ExtrusionCrossSection=frame_xsec  ExtrusionCrossSectionUnits=cm  ExtrusionLength=T  ExtrusionLengthUnits=cm  PolygonNumSides=3  PolygonOuterRadius=1  PolygonOuterRadiusUnits=m  ExtGeomFileType=STL  ExtGeomFileUnits=m  RevolutionCrossSection=[1 1; 1 -1; 2 -1; 2 1]  RevolutionCrossSectionUnits=m  RevolutionExtent=Full  RevolutionAngle=180  RevolutionAngleUnits=deg
  UL XForm : sm_lib/Frames and Transforms/Rigid Transform  TranslationMethod=Cartesian  TranslationStandardOffset=0  TranslationLengthUnit=cm  TranslationStandardAxis=+Z  TranslationCartesianOffset=[nwc 0]  TranslationROffset=0  TranslationROffsetUnits=m  TranslationZOffset=0  TranslationZOffsetUnits=m  TranslationThetaOffset=0  TranslationThetaOffsetUnits=deg  RotationMethod=None  RotationAngleUnits=deg  RotationStandardAxis=+Z  RotationAngle=0  RotationArbitraryAxis=[0 0 1]  FollAlignAxisA=+X  BaseAlignAxisA=-X  FollAlignAxisB=+Y  BaseAlignAxisB=-Y  RotationSequenceAxes=FollowerAxes  RotationSequence=XYX  RotationSequenceAngles=[0 0 0]  RotationSequenceAnglesUnits=deg  RotationMatrix=[1 0 0; 0 1 0; 0 0 1]
  UR XForm : sm_lib/Frames and Transforms/Rigid Transform  TranslationMethod=Cartesian  TranslationStandardOffset=0  TranslationLengthUnit=cm  TranslationStandardAxis=+Z  TranslationCartesianOffset=[nec 0]  TranslationROffset=0  TranslationROffsetUnits=m  TranslationZOffset=0  TranslationZOffsetUnits=m  TranslationThetaOffset=0  TranslationThetaOffsetUnits=deg  RotationMethod=None  RotationAngleUnits=deg  RotationStandardAxis=+Z  RotationAngle=0  RotationArbitraryAxis=[0 0 1]  FollAlignAxisA=+X  BaseAlignAxisA=+Y  FollAlignAxisB=+Y  BaseAlignAxisB=+Z  RotationSequenceAxes=FollowerAxes  RotationSequence=XYX  RotationSequenceAngles=[0 0 0]  RotationSequenceAnglesUnits=deg  RotationMatrix=[1 0 0; 0 1 0; 0 0 1]
  UL : PMIOPort  Port=1  Side=Left
  DL : PMIOPort  Port=2  Side=Left
  DR : PMIOPort  Port=3  Side=Left
  UR : PMIOPort  Port=4  Side=Left
  connections:
  Frame/RConn1 -- UL XForm/LConn1 -- DL XForm/LConn1 -- DR XForm/LConn1 -- UR XForm/LConn1
  UR XForm/RConn1 -- UR/RConn1
  DL XForm/RConn1 -- DL/RConn1
  UL XForm/RConn1 -- UL/RConn1
  DR XForm/RConn1 -- DR/RConn1

== system VehicleDynamics3D/FrontSuspension/Chassis Assembly/Load ==
  Chassis Load : sm_lib/Body Elements/Solid  InertiaType=PointMass  Mass=Load  MassUnits=kg  CenterOfMass=[0 0 0]  CenterOfMassUnits=m  MomentsOfInertia=[1 1 1]  MomentsOfInertiaUnits=kg*m^2  ProductsOfInertia=[0 0 0]  ProductsOfInertiaUnits=kg*m^2  DensityBased=off  Density=1000  DensityUnits=kg/(m^3)  DoExposeReferenceFrame=on  SerializedFrames=<Frames/>  GraphicType=FromGeometry  MarkerShape=Sphere  MarkerSize=10  MarkerSizeUnits=m  GraphicVisPropType=SimpleVisualProperties  GraphicDiffuseColor=[0.6 0.0 0.0]  GraphicSpecularColor=[0.5 0.5 0.5 1.0]  GraphicAmbientColor=[0.15 0.15 0.15 1.0]  GraphicEmissiveColor=[0.0 0.0 0.0 1.0]  GraphicShininess=75  GraphicOpacity=1.0  GeometryShape=Brick  RectangleSize=[1 1]  RectangleSizeUnits=m  BrickDimensions=[5 5 5]  BrickDimensionUnits=cm  CylinderRadius=1  CylinderRadiusUnits=m  CylinderLength=1  CylinderLengthUnits=m  SphereRadius=1  SphereRadiusUnits=m  EllipsoidRadii=[1 1 1]  EllipsoidRadiiUnits=m  ExtrusionCrossSection=[1 1; -1 1; -1 -1; 1 -1]  ExtrusionCrossSectionUnits=m  ExtrusionLength=1  ExtrusionLengthUnits=m  PolygonNumSides=3  PolygonOuterRadius=1  PolygonOuterRadiusUnits=m  ExtGeomFileType=STL  ExtGeomFileUnits=m  RevolutionCrossSection=[1 1; 1 -1; 2 -1; 2 1]  RevolutionCrossSectionUnits=m  RevolutionExtent=Full  RevolutionAngle=180  RevolutionAngleUnits=deg
  Chassis Load XForm : sm_lib/Frames and Transforms/Rigid Transform  TranslationMethod=StandardAxis  TranslationStandardOffset=15  TranslationLengthUnit=cm  TranslationStandardAxis=+X  TranslationCartesianOffset=[0 0 0]  TranslationROffset=0  TranslationROffsetUnits=m  TranslationZOffset=0  TranslationZOffsetUnits=m  TranslationThetaOffset=0  TranslationThetaOffsetUnits=deg  RotationMethod=None  RotationAngleUnits=deg  RotationStandardAxis=+Z  RotationAngle=0  RotationArbitraryAxis=[0 0 1]  FollAlignAxisA=+X  BaseAlignAxisA=+Y  FollAlignAxisB=+Y  BaseAlignAxisB=+Z  RotationSequenceAxes=FollowerAxes  RotationSequence=XYX  RotationSequenceAngles=[0 0 0]  RotationSequenceAnglesUnits=deg  RotationMatrix=[1 0 0; 0 1 0; 0 0 1]
  L : PMIOPort  Port=1  Side=Right
  connections:
  Chassis Load XForm/LConn1 -- L/RConn1
  Chassis Load/RConn1 -- Chassis Load XForm/RConn1
